simulink model "abslut50_fixpt8_19"  (R2021b)
settings: Solver=VariableStepAuto  StartTime=0.0  StopTime=99  RelTol=1e-3
undefined symbols (not defined in the file or in its folder): figd2104, xcu250
libraries: hdlBasic x4666, vmcUtilities x1
(part 15 of 15)

== matlab function abslut50_fixpt8_19/MATLAB Function2 ==
  data: x input; out output; y input
function out = fcn(x,y)
out = sqrt(x.^2 + y.^2);

== matlab function abslut50_fixpt8_19/MATLAB Function3 ==
  data: u8 input; u9 input; u10 input; u11 input; u12 input; u13 input; u14 input; u15 input; u16 input; u17 input; u18 input; u19 input; y8 output; y9 output; y10 output; y11 output; y12 output; y13 output; y14 output; y15 output; x input; y16 output; y17 output; y18 output; y19 output
function [y8,y9,y10,y11,y12,y13,y14,y15,y16,y17,y18,y19] = fcn(u8,u9,u10,u11,u12,u13,u14,u15,u16,u17,u18,u19,x)
y8 = (u8 - x).^2;
y9 = (u9 - x).^2;
y10 = (u10 - x).^2;
y11 = (u11 - x).^2;
y12 = (u12 - x).^2;
y13 = (u13 - x).^2;
y14 = (u14 - x).^2;
y15 = (u15 - x).^2;
y16 = (u16 - x).^2;
y17 = (u17 - x).^2;
y18 = (u18 - x).^2;
y19 = (u19 - x).^2;
